simulink model "hdv_hydroelectropowertrain_model"  (R2023b)
settings: Solver=ode1be  StartTime=0.0  StopTime=simulation_length  FixedStep=tsample  MaxStep=tsample
values from neighbouring files (symbols this model uses):
  alpha = 35    [init_model.m]
  Apump = [0 1; 0 0]    [init_model.m]
  available_torque = torque_base+torque_friction_base    [init_model.m]
  Bpump = [0 1]'    [init_model.m]
  btheta_shaft = 2e2    (= 200)    [init_model.m]
  C1 = 10    [init_model.m]
  consumption = [consumption_1, consumption_2, consumption_3, consumption_4,          consumption_5, consumption_6, consumption_7, consumption_8,          consumption_9, consumption_10, consumption_11, consumption_12,          consumption_13, consumption_14, consumption_15, consumption_16          ]    [ic_engine_data.m]
  Cpump = [k 0]    [init_model.m]
  dp_lim = 400    [init_model.m]
  E0 = 3.685    [init_model.m]
  E1 = 0.2156    [init_model.m]
  E2 = 0    [init_model.m]
  E3 = 0    [init_model.m]
  E_1 = -1.031    [init_model.m]
  Elog = -0.05    [init_model.m]
  eta_v_m = 0.98    [init_model.m]
  eta_v_p = 0.97    [init_model.m]
  ki_dp_comp = 1/dp_lim    (= 0.0025)    [init_model.m]
  ki_te_comp = 2/te_lim    [init_model.m]
  kp_ctrl_m = 1    [init_model.m]
  kp_dp_comp = 0.5/dp_lim    (= 0.00125)    [init_model.m]
  kp_te_comp = 1/te_lim    [init_model.m]
  Kpump = acker(Apump,Bpump,poles)    [init_model.m]
  load_blade_enable = 0    [init_model.m]
  Lpump = acker(Apump',Cpump',pole_so)'    [init_model.m]
  M = 125    [init_model.m]
  Ncell = 185    [init_model.m]
  Npump = -1/(Cpump*inv(Apump-Bpump*Kpump)*Bpump)    [init_model.m]
  omega_e_rpm_ref = 1700    [init_model.m]
  omega_l_max_rpm = omega_l_max/(2*pi)*60    (= 50.3075969543)    [init_model.m]
  q1Kalman = tsample^2*1e-2    (= 1e-08)    [init_model.m]
  q2Kalman = tsample^1*1e-1    (= 0.0001)    [init_model.m]
  q3Kalman = 0    [init_model.m]
  Qhr = 400    [init_model.m]
  R0 = 0.015    [init_model.m]
  R1 = 0.015    [init_model.m]
  R_tg = 1.16/2    (= 0.58)    [init_model.m]
  rKalman = 1    [init_model.m]
  rpm_base = [620 700 800 900 1000 1100 1200 1300 1400 1500 1600 1700 1800      1900 2000 2100]    [ic_engine_data.m]
  rpm_consumption = rpm_base    [ic_engine_data.m]
  simulation_length = 245    [init_model.m]
  tau_load = 75e3    (= 75000)    [init_model.m]
  tau_load_max = 1600*41.4    (= 66240)    [init_model.m]
  Tc = tsample    (= 0.001)    [init_model.m]
  torque_base = [max(torque_16_data) max(torque_15_data) max(torque_14_data)      max(torque_13_data) max(torque_12_data) max(torque_11_data)      max(torque_10_data) max(torque_9_data) max(torque_8_data)      max(torque_7_data) max(torque_6_data) max(torque_5_data)      max(torque_4_data) max(torque_3_data) max(torque_2_data)      max(torque_1_data)]    [ic_engine_data.m]
  torque_consumption = torque_reference    [ic_engine_data.m]
  torque_friction_base = -(rpm_base./60*2*pi)*0.25-(rpm_base./60*2*pi).^2*5.2e-4    [ic_engine_data.m]
  tsample = 1e-3    (= 0.001)    [init_model.m]
  v_track1_ref = 8    [init_model.m]
  v_track2_ref = 8    [init_model.m]
  valve_mmorifice_max = 2.75    [init_model.m]
  xv_m_max = 1.2    [init_model.m]
undefined symbols (not defined in the file or in its folder): magnitude
libraries: fl_lib x381, nesl_utility x162, linear_swashplate_ctrl_lib x8, flexshaft_lib x5, bichamber_piston_lib x5, variable_displacement_motor_lib x4, variable_displacement_pump_lib x4, fixed_displacement_pump_lib x4, relief_valve_lib x4, inverse_shuttle_valve_lib x4, hydrostatic_threeway_valve_bichamber_piston_lib x4, hydrostatic_fourway_valve_bichamber_piston_lib x4
(part 5 of 9)

== system hdv_hydroelectropowertrain_model/PR776_powertrain/Hydrostatic_powertrain/driveine_LD2/pressure_charge_system_LD ==
  Hydraulic Flow Rate Sensor : fl_lib/Hydraulic/Hydraulic Sensors/Hydraulic Flow Rate Sensor
  Hydraulic Flow Rate Sensor1 : fl_lib/Hydraulic/Hydraulic Sensors/Hydraulic Flow Rate Sensor
  Hydraulic Pressure Sensor{1..4} (4 alike) : fl_lib/Hydraulic/Hydraulic Sensors/Hydraulic Pressure Sensor
  Hydraulic Reference1 : fl_lib/Hydraulic/Hydraulic Elements/Hydraulic Reference
  Hydraulic Reference2 : fl_lib/Hydraulic/Hydraulic Elements/Hydraulic Reference
  Hydraulic Reference3 : fl_lib/Hydraulic/Hydraulic Elements/Hydraulic Reference
  Mux : Mux  Inputs=2
  PS-Simulink Converter : nesl_utility/PS-Simulink Converter  PhysicalDomain=network_engine_domain  SubClassName=ps_output  LeftPortType=input  RightPortType=output  PseudoPeriodic=off  Frequencies=[]  VectorFormat=1-D array  Unit=l/min  AffineConversion=on
  PS-Simulink Converter{1..3,5} (4 alike) : nesl_utility/PS-Simulink Converter  PhysicalDomain=network_engine_domain  SubClassName=ps_output  LeftPortType=input  RightPortType=output  PseudoPeriodic=off  Frequencies=[]  VectorFormat=1-D array  Unit=bar  AffineConversion=on
  PS-Simulink Converter4 : nesl_utility/PS-Simulink Converter  PhysicalDomain=network_engine_domain  SubClassName=ps_output  LeftPortType=input  RightPortType=output  PseudoPeriodic=off  Frequencies=[]  VectorFormat=1-D array  Unit=l/min  AffineConversion=on
  Scope1 : Scope  NumInputPorts=2
  Scope2 : Scope  NumInputPorts=2
  Scope3 : Scope  NumInputPorts=2
  Subsystem : Subsystem
  hydro_check_valve1 : Subsystem
      settings: PortSchema="{\"entries\":[{\"content\":{\"sides\":[{\"content\":{\"connectorIds\":[]},\"type\":\"ConnectorPlacement.EquallySpacedRectSide\",\"uuid\":\"a69fbb91-2279-4dfd-af6f-16497d5f1538\"},{\"content\":{\"connectorIds\":[],\"side\":\"RIGHT\"},\"type\":\"ConnectorPlacement.EquallySpacedRectSide\",\"uuid\":\"52e95d44-b7af-4ccc-8556-a2abd2e724e0\"},{\"content\":{\"connectorIds\":[\"LConn1\"],\"side\":\"TOP\"},\"type\":\"ConnectorPlacement.EquallySpacedRectSide\",\"uuid\":\"2d8c071e-4cd0-4b83-8d45-c175cb858754\"},{\"content\":{\"connectorIds\":[\"RConn1\"],\"side\":\"BOTTOM\"},\"type\":\"ConnectorPlacement.EquallySpacedRectSide\",\"uuid\":\"1baec9dc-757c-4f21-904a-6fc08de72ce1\"}]},\"type\":\"ConnectorPlacement.EquallySpacedConnector\",\"uuid\":\"76990e53-6cb0-4bfe-8c9e-427c41b785f2\"}],\"packageUris\":[\"http://schema.mathworks.com/mf0/Connector/19700101\"],\"version\":\"1.0\"}"
  hydro_check_valve2 : Subsystem
      settings: PortSchema="{\"entries\":[{\"content\":{\"sides\":[{\"content\":{\"connectorIds\":[]},\"type\":\"ConnectorPlacement.EquallySpacedRectSide\",\"uuid\":\"a69fbb91-2279-4dfd-af6f-16497d5f1538\"},{\"content\":{\"connectorIds\":[],\"side\":\"RIGHT\"},\"type\":\"ConnectorPlacement.EquallySpacedRectSide\",\"uuid\":\"52e95d44-b7af-4ccc-8556-a2abd2e724e0\"},{\"content\":{\"connectorIds\":[\"LConn1\"],\"side\":\"TOP\"},\"type\":\"ConnectorPlacement.EquallySpacedRectSide\",\"uuid\":\"2d8c071e-4cd0-4b83-8d45-c175cb858754\"},{\"content\":{\"connectorIds\":[\"RConn1\"],\"side\":\"BOTTOM\"},\"type\":\"ConnectorPlacement.EquallySpacedRectSide\",\"uuid\":\"1baec9dc-757c-4f21-904a-6fc08de72ce1\"}]},\"type\":\"ConnectorPlacement.EquallySpacedConnector\",\"uuid\":\"76990e53-6cb0-4bfe-8c9e-427c41b785f2\"}],\"packageUris\":[\"http://schema.mathworks.com/mf0/Connector/19700101\"],\"version\":\"1.0\"}"
  inverse shuttle valve : inverse_shuttle_valve_lib/inverse shuttle valve  pnom=32 bar  dp_crack=0 bar  dp_reg=0 bar  x_rv_max=2 mm  a0=(2*pi*10)^2 1/s^2  a1=2*2*pi*10 1/s  leak=5e-12 m^3/s/Pa  qA_specify=off  qA_priority=None  qA=0 m^3/s  qA_nominal_specify=off  qA_nominal_unit=m^3/s  qA_nominal_value=1  qB_specify=off  qB_priority=None  qB=0 m^3/s  qB_nominal_specify=off  qB_nominal_unit=m^3/s  qB_nominal_value=1  qP_specify=off  qP_priority=None  qP=0 m^3/s  qP_nominal_specify=off  qP_nominal_unit=m^3/s  qP_nominal_value=1  dp_specify=off  dp_priority=None  dp=0 Pa  dp_nominal_specify=off  dp_nominal_unit=Pa  dp_nominal_value=1  dpAP_specify=off  dpAP_priority=None  dpAP=0 Pa  dpAP_nominal_specify=off  dpAP_nominal_unit=Pa  dpAP_nominal_value=1  dpBP_specify=off  dpBP_priority=None  dpBP=0 Pa  dpBP_nominal_specify=off  dpBP_nominal_unit=Pa  dpBP_nominal_value=1  x_rv_AP_specify=off  x_rv_AP_priority=None  x_rv_AP=0 m  x_rv_AP_nominal_specify=off  x_rv_AP_nominal_unit=m  x_rv_AP_nominal_value=1  x_rv_BP_specify=off  x_rv_BP_priority=None  x_rv_BP=0 m  x_rv_BP_nominal_specify=off  x_rv_BP_nominal_unit=m  x_rv_BP_nominal_value=1  x_rv_AP_flt_specify=off  x_rv_AP_flt_priority=None  x_rv_AP_flt=0 m  x_rv_AP_flt_nominal_specify=off  x_rv_AP_flt_nominal_unit=m  x_rv_AP_flt_nominal_value=1  x_rv_BP_flt_specify=off  x_rv_BP_flt_priority=None  x_rv_BP_flt=0 m  x_rv_BP_flt_nominal_specify=off  x_rv_BP_flt_nominal_unit=m  x_rv_BP_flt_nominal_value=1
      settings: InternalSimscapePortConfiguration="{\"Bottom\":[],\"Left\":[{\"id\":\"cA\",\"label\":\"cA\",\"type\":\"foundation.hydraulic.hydraulic\"},{\"id\":\"cB\",\"label\":\"cB\",\"type\":\"foundation.hydraulic.hydraulic\"}],\"Right\":[{\"id\":\"cP\",\"label\":\"cP\",\"type\":\"foundation.hydraulic.hydraulic\"}],\"Top\":[]}"
  A : PMIOPort  Side=Left
  B : PMIOPort  Port=2  Side=Right
  D : PMIOPort  Port=3  Side=Right
  wires:
  PS-Simulink Converter2/1 -> Mux/2  "pA"
  PS-Simulink Converter1/1 -> Mux/1  "pB"
  Mux/1 -> Scope1/1
  PS-Simulink Converter/1 -> Scope2/1, Scope1/2  "qcharge"
  PS-Simulink Converter3/1 -> Scope2/2  "pCharge"
  PS-Simulink Converter4/1 -> Scope3/1  "qT_ishuttle"
  PS-Simulink Converter5/1 -> Scope3/2  "dp"
  connections:
  inverse shuttle valve/RConn1 -- Hydraulic Flow Rate Sensor1/LConn1
  hydro_check_valve2/LConn1 -- Hydraulic Flow Rate Sensor/RConn2 -- hydro_check_valve1/LConn1
  hydro_check_valve1/RConn1 -- inverse shuttle valve/LConn1 -- A/RConn1 -- Hydraulic Pressure Sensor2/LConn1 -- Hydraulic Pressure Sensor4/LConn1
  hydro_check_valve2/RConn1 -- inverse shuttle valve/LConn2 -- B/RConn1 -- Hydraulic Pressure Sensor1/LConn1 -- Hydraulic Pressure Sensor4/RConn1
  Hydraulic Pressure Sensor2/RConn1 -- Hydraulic Reference1/LConn1 -- Hydraulic Pressure Sensor1/RConn1
  Hydraulic Pressure Sensor1/RConn2 -- PS-Simulink Converter1/LConn1
  Hydraulic Pressure Sensor2/RConn2 -- PS-Simulink Converter2/LConn1
  Hydraulic Flow Rate Sensor/RConn1 -- PS-Simulink Converter/LConn1
  Hydraulic Pressure Sensor3/LConn1 -- Subsystem/RConn1 -- Hydraulic Flow Rate Sensor/LConn1
  Subsystem/LConn1 -- D/RConn1
  Hydraulic Pressure Sensor3/RConn2 -- PS-Simulink Converter3/LConn1
  Hydraulic Reference2/LConn1 -- Hydraulic Pressure Sensor3/RConn1
  Hydraulic Flow Rate Sensor1/RConn2 -- Hydraulic Reference3/LConn1
  Hydraulic Flow Rate Sensor1/RConn1 -- PS-Simulink Converter4/LConn1
  PS-Simulink Converter5/LConn1 -- Hydraulic Pressure Sensor4/RConn2

== system hdv_hydroelectropowertrain_model/PR776_powertrain/Hydrostatic_powertrain/driveine_LD2/vd_ctrl_motor_LD ==
  vd_ref : Inport
  Linear swashplate ctrl2 : linear_swashplate_ctrl_lib/Linear swashplate ctrl  Commented=on  a12=1 1/s  b2=1 1/m/s  k1=100 m  k2=20.5 m  N=5 m  kv=20  xv_specify=off  xv_priority=None  xv=0 m  xv_nominal_specify=off  xv_nominal_unit=m  xv_nominal_value=1  D1_specify=off  D1_priority=None  D1=0  D1_nominal_specify=off  D1_nominal_unit=1  D1_nominal_value=1  D2_specify=off  D2_priority=None  D2=0  D2_nominal_specify=off  D2_nominal_unit=1  D2_nominal_value=1
      settings: InternalSimscapePortConfiguration="{\"Bottom\":[],\"Left\":[{\"id\":\"D_ref\",\"label\":\"Dref\",\"type\":\"input\"}],\"Right\":[{\"id\":\"Dout\",\"label\":\"Dout\",\"type\":\"output\"}],\"Top\":[]}"
  PS-Simulink Converter : nesl_utility/PS-Simulink Converter  PhysicalDomain=network_engine_domain  SubClassName=ps_output  LeftPortType=input  RightPortType=output  PseudoPeriodic=off  Frequencies=[]  VectorFormat=1-D array  Unit=inherit  AffineConversion=off
  Scope : Scope  NumInputPorts=2
  Simulink-PS Converter3 : nesl_utility/Simulink-PS Converter  Commented=on  PhysicalDomain=network_engine_domain  SubClassName=ps_input  LeftPortType=input  RightPortType=output  PseudoPeriodic=off  Frequencies=[]  NoiseDistribution=none  NoiseParameters=[]  Unit=1  AffineConversion=off  FilteringAndDerivatives=provide  SimscapeFilterOrder=1  InputFilterTimeConstant=0.001  UdotUserProvided=0
  hose3 : Subsystem
  servo motor LD : Subsystem
  vd : PMIOPort  Side=Right
  pS : PMIOPort  Port=2  Side=Left
  pT : PMIOPort  Port=3  Side=Left
  wires:
  vd_ref/1 -> Simulink-PS Converter3/1, Scope/1, servo motor LD/1(displacement reference pu)
  PS-Simulink Converter/1 -> Scope/2
  connections:
  vd/RConn1 -- PS-Simulink Converter/LConn1 -- servo motor LD/RConn1
  hose3/RConn2 -- servo motor LD/LConn2
  hose3/RConn1 -- servo motor LD/LConn1
  pT/RConn1 -- hose3/LConn2
  pS/RConn1 -- hose3/LConn1
  Simulink-PS Converter3/RConn1 -- Linear swashplate ctrl2/LConn1

== system hdv_hydroelectropowertrain_model/PR776_powertrain/Hydrostatic_powertrain/driveine_LD2/vd_ctrl_pump_LD ==
  vd_ref : Inport
  Linear swashplate ctrl2 : linear_swashplate_ctrl_lib/Linear swashplate ctrl  Commented=on  a12=1 1/s  b2=1 1/m/s  k1=100 m  k2=20.5 m  N=5 m  kv=20  xv_specify=off  xv_priority=None  xv=0 m  xv_nominal_specify=off  xv_nominal_unit=m  xv_nominal_value=1  D1_specify=off  D1_priority=None  D1=0  D1_nominal_specify=off  D1_nominal_unit=1  D1_nominal_value=1  D2_specify=off  D2_priority=None  D2=0  D2_nominal_specify=off  D2_nominal_unit=1  D2_nominal_value=1
      settings: InternalSimscapePortConfiguration="{\"Bottom\":[],\"Left\":[{\"id\":\"D_ref\",\"label\":\"Dref\",\"type\":\"input\"}],\"Right\":[{\"id\":\"Dout\",\"label\":\"Dout\",\"type\":\"output\"}],\"Top\":[]}"
  Simulink-PS Converter3 : nesl_utility/Simulink-PS Converter  Commented=on  PhysicalDomain=network_engine_domain  SubClassName=ps_input  LeftPortType=input  RightPortType=output  PseudoPeriodic=off  Frequencies=[]  NoiseDistribution=none  NoiseParameters=[]  Unit=1  AffineConversion=off  FilteringAndDerivatives=provide  SimscapeFilterOrder=1  InputFilterTimeConstant=0.001  UdotUserProvided=0
  hose3 : Subsystem
  servo pump RD : Subsystem
  vd : PMIOPort  Side=Right
  pS : PMIOPort  Port=2  Side=Left
  pT : PMIOPort  Port=3  Side=Left
  wires:
  vd_ref/1 -> servo pump RD/1(displacement reference pu), Simulink-PS Converter3/1
  connections:
  servo pump RD/RConn1 -- vd/RConn1
  Simulink-PS Converter3/RConn1 -- Linear swashplate ctrl2/LConn1
  servo pump RD/LConn2 -- hose3/RConn2
  servo pump RD/LConn1 -- hose3/RConn1
  pS/RConn1 -- hose3/LConn1
  pT/RConn1 -- hose3/LConn2

== system hdv_hydroelectropowertrain_model/PR776_powertrain/Hydrostatic_powertrain/driveine_RD1/pressure_charge_system_RD ==
  Hydraulic Flow Rate Sensor : fl_lib/Hydraulic/Hydraulic Sensors/Hydraulic Flow Rate Sensor
  Hydraulic Flow Rate Sensor1 : fl_lib/Hydraulic/Hydraulic Sensors/Hydraulic Flow Rate Sensor
  Hydraulic Pressure Sensor{1..4} (4 alike) : fl_lib/Hydraulic/Hydraulic Sensors/Hydraulic Pressure Sensor
  Hydraulic Reference1 : fl_lib/Hydraulic/Hydraulic Elements/Hydraulic Reference
  Hydraulic Reference2 : fl_lib/Hydraulic/Hydraulic Elements/Hydraulic Reference
  Hydraulic Reference3 : fl_lib/Hydraulic/Hydraulic Elements/Hydraulic Reference
  Mux : Mux  Inputs=2
  PS-Simulink Converter : nesl_utility/PS-Simulink Converter  PhysicalDomain=network_engine_domain  SubClassName=ps_output  LeftPortType=input  RightPortType=output  PseudoPeriodic=off  Frequencies=[]  VectorFormat=1-D array  Unit=l/min  AffineConversion=on
  PS-Simulink Converter{1..3,5} (4 alike) : nesl_utility/PS-Simulink Converter  PhysicalDomain=network_engine_domain  SubClassName=ps_output  LeftPortType=input  RightPortType=output  PseudoPeriodic=off  Frequencies=[]  VectorFormat=1-D array  Unit=bar  AffineConversion=on
  PS-Simulink Converter4 : nesl_utility/PS-Simulink Converter  PhysicalDomain=network_engine_domain  SubClassName=ps_output  LeftPortType=input  RightPortType=output  PseudoPeriodic=off  Frequencies=[]  VectorFormat=1-D array  Unit=l/min  AffineConversion=on
  Scope1 : Scope  NumInputPorts=2
  Scope2 : Scope  NumInputPorts=2
  Subsystem : Subsystem
  hydro_check_valve1 : Subsystem
      settings: PortSchema="{\"entries\":[{\"content\":{\"sides\":[{\"content\":{\"connectorIds\":[]},\"type\":\"ConnectorPlacement.EquallySpacedRectSide\",\"uuid\":\"a69fbb91-2279-4dfd-af6f-16497d5f1538\"},{\"content\":{\"connectorIds\":[],\"side\":\"RIGHT\"},\"type\":\"ConnectorPlacement.EquallySpacedRectSide\",\"uuid\":\"52e95d44-b7af-4ccc-8556-a2abd2e724e0\"},{\"content\":{\"connectorIds\":[\"LConn1\"],\"side\":\"TOP\"},\"type\":\"ConnectorPlacement.EquallySpacedRectSide\",\"uuid\":\"2d8c071e-4cd0-4b83-8d45-c175cb858754\"},{\"content\":{\"connectorIds\":[\"RConn1\"],\"side\":\"BOTTOM\"},\"type\":\"ConnectorPlacement.EquallySpacedRectSide\",\"uuid\":\"1baec9dc-757c-4f21-904a-6fc08de72ce1\"}]},\"type\":\"ConnectorPlacement.EquallySpacedConnector\",\"uuid\":\"76990e53-6cb0-4bfe-8c9e-427c41b785f2\"}],\"packageUris\":[\"http://schema.mathworks.com/mf0/Connector/19700101\"],\"version\":\"1.0\"}"
  hydro_check_valve2 : Subsystem
      settings: PortSchema="{\"entries\":[{\"content\":{\"sides\":[{\"content\":{\"connectorIds\":[]},\"type\":\"ConnectorPlacement.EquallySpacedRectSide\",\"uuid\":\"a69fbb91-2279-4dfd-af6f-16497d5f1538\"},{\"content\":{\"connectorIds\":[],\"side\":\"RIGHT\"},\"type\":\"ConnectorPlacement.EquallySpacedRectSide\",\"uuid\":\"52e95d44-b7af-4ccc-8556-a2abd2e724e0\"},{\"content\":{\"connectorIds\":[\"LConn1\"],\"side\":\"TOP\"},\"type\":\"ConnectorPlacement.EquallySpacedRectSide\",\"uuid\":\"2d8c071e-4cd0-4b83-8d45-c175cb858754\"},{\"content\":{\"connectorIds\":[\"RConn1\"],\"side\":\"BOTTOM\"},\"type\":\"ConnectorPlacement.EquallySpacedRectSide\",\"uuid\":\"1baec9dc-757c-4f21-904a-6fc08de72ce1\"}]},\"type\":\"ConnectorPlacement.EquallySpacedConnector\",\"uuid\":\"76990e53-6cb0-4bfe-8c9e-427c41b785f2\"}],\"packageUris\":[\"http://schema.mathworks.com/mf0/Connector/19700101\"],\"version\":\"1.0\"}"
  inverse shuttle valve : inverse_shuttle_valve_lib/inverse shuttle valve  pnom=32 bar  dp_crack=0 bar  dp_reg=0 bar  x_rv_max=2 mm  a0=(2*pi*10)^2 1/s^2  a1=2*2*pi*10 1/s  leak=5e-12 m^3/s/Pa  qA_specify=off  qA_priority=None  qA=0 m^3/s  qA_nominal_specify=off  qA_nominal_unit=m^3/s  qA_nominal_value=1  qB_specify=off  qB_priority=None  qB=0 m^3/s  qB_nominal_specify=off  qB_nominal_unit=m^3/s  qB_nominal_value=1  qP_specify=off  qP_priority=None  qP=0 m^3/s  qP_nominal_specify=off  qP_nominal_unit=m^3/s  qP_nominal_value=1  dp_specify=off  dp_priority=None  dp=0 Pa  dp_nominal_specify=off  dp_nominal_unit=Pa  dp_nominal_value=1  dpAP_specify=off  dpAP_priority=None  dpAP=0 Pa  dpAP_nominal_specify=off  dpAP_nominal_unit=Pa  dpAP_nominal_value=1  dpBP_specify=off  dpBP_priority=None  dpBP=0 Pa  dpBP_nominal_specify=off  dpBP_nominal_unit=Pa  dpBP_nominal_value=1  x_rv_AP_specify=off  x_rv_AP_priority=None  x_rv_AP=0 m  x_rv_AP_nominal_specify=off  x_rv_AP_nominal_unit=m  x_rv_AP_nominal_value=1  x_rv_BP_specify=off  x_rv_BP_priority=None  x_rv_BP=0 m  x_rv_BP_nominal_specify=off  x_rv_BP_nominal_unit=m  x_rv_BP_nominal_value=1  x_rv_AP_flt_specify=off  x_rv_AP_flt_priority=None  x_rv_AP_flt=0 m  x_rv_AP_flt_nominal_specify=off  x_rv_AP_flt_nominal_unit=m  x_rv_AP_flt_nominal_value=1  x_rv_BP_flt_specify=off  x_rv_BP_flt_priority=None  x_rv_BP_flt=0 m  x_rv_BP_flt_nominal_specify=off  x_rv_BP_flt_nominal_unit=m  x_rv_BP_flt_nominal_value=1
      settings: InternalSimscapePortConfiguration="{\"Bottom\":[],\"Left\":[{\"id\":\"cA\",\"label\":\"cA\",\"type\":\"foundation.hydraulic.hydraulic\"},{\"id\":\"cB\",\"label\":\"cB\",\"type\":\"foundation.hydraulic.hydraulic\"}],\"Right\":[{\"id\":\"cP\",\"label\":\"cP\",\"type\":\"foundation.hydraulic.hydraulic\"}],\"Top\":[]}"
  qt_ishuttle/dp : Scope  NumInputPorts=2
  A : PMIOPort  Side=Left
  B : PMIOPort  Port=2  Side=Right
  D : PMIOPort  Port=3  Side=Right
  wires:
  PS-Simulink Converter2/1 -> Mux/2  "pA"
  PS-Simulink Converter1/1 -> Mux/1  "pB"
  Mux/1 -> Scope1/1
  PS-Simulink Converter/1 -> Scope1/2, Scope2/1  "qcharge"
  PS-Simulink Converter3/1 -> Scope2/2  "pCharge"
  PS-Simulink Converter4/1 -> qt_ishuttle/dp/1  "qt_ishuttle"
  PS-Simulink Converter5/1 -> qt_ishuttle/dp/2  "dp"
  connections:
  hydro_check_valve2/LConn1 -- Hydraulic Flow Rate Sensor/RConn2 -- hydro_check_valve1/LConn1
  A/RConn1 -- Hydraulic Pressure Sensor4/LConn1 -- inverse shuttle valve/LConn1 -- hydro_check_valve1/RConn1 -- Hydraulic Pressure Sensor2/LConn1
  B/RConn1 -- Hydraulic Pressure Sensor4/RConn1 -- inverse shuttle valve/LConn2 -- hydro_check_valve2/RConn1 -- Hydraulic Pressure Sensor1/LConn1
  Hydraulic Pressure Sensor2/RConn1 -- Hydraulic Reference1/LConn1 -- Hydraulic Pressure Sensor1/RConn1
  Hydraulic Pressure Sensor1/RConn2 -- PS-Simulink Converter1/LConn1
  Hydraulic Pressure Sensor2/RConn2 -- PS-Simulink Converter2/LConn1
  Hydraulic Flow Rate Sensor/RConn1 -- PS-Simulink Converter/LConn1
  Hydraulic Pressure Sensor3/LConn1 -- Subsystem/RConn1 -- Hydraulic Flow Rate Sensor/LConn1
  Subsystem/LConn1 -- D/RConn1
  Hydraulic Pressure Sensor3/RConn2 -- PS-Simulink Converter3/LConn1
  Hydraulic Reference2/LConn1 -- Hydraulic Pressure Sensor3/RConn1
  Hydraulic Flow Rate Sensor1/RConn2 -- Hydraulic Reference3/LConn1
  Hydraulic Flow Rate Sensor1/RConn1 -- PS-Simulink Converter4/LConn1
  PS-Simulink Converter5/LConn1 -- Hydraulic Pressure Sensor4/RConn2
  inverse shuttle valve/RConn1 -- Hydraulic Flow Rate Sensor1/LConn1

== system hdv_hydroelectropowertrain_model/PR776_powertrain/Hydrostatic_powertrain/driveine_RD1/vd_ctrl_motor_RD ==
  vd_ref : Inport
  Linear swashplate ctrl2 : linear_swashplate_ctrl_lib/Linear swashplate ctrl  Commented=on  a12=1 1/s  b2=1 1/m/s  k1=100 m  k2=20.5 m  N=5 m  kv=20  xv_specify=off  xv_priority=None  xv=0 m  xv_nominal_specify=off  xv_nominal_unit=m  xv_nominal_value=1  D1_specify=off  D1_priority=None  D1=0  D1_nominal_specify=off  D1_nominal_unit=1  D1_nominal_value=1  D2_specify=off  D2_priority=None  D2=0  D2_nominal_specify=off  D2_nominal_unit=1  D2_nominal_value=1
      settings: InternalSimscapePortConfiguration="{\"Bottom\":[],\"Left\":[{\"id\":\"D_ref\",\"label\":\"Dref\",\"type\":\"input\"}],\"Right\":[{\"id\":\"Dout\",\"label\":\"Dout\",\"type\":\"output\"}],\"Top\":[]}"
  PS-Simulink Converter : nesl_utility/PS-Simulink Converter  PhysicalDomain=network_engine_domain  SubClassName=ps_output  LeftPortType=input  RightPortType=output  PseudoPeriodic=off  Frequencies=[]  VectorFormat=1-D array  Unit=inherit  AffineConversion=off
  Scope : Scope  NumInputPorts=2
  Simulink-PS Converter3 : nesl_utility/Simulink-PS Converter  Commented=on  PhysicalDomain=network_engine_domain  SubClassName=ps_input  LeftPortType=input  RightPortType=output  PseudoPeriodic=off  Frequencies=[]  NoiseDistribution=none  NoiseParameters=[]  Unit=1  AffineConversion=off  FilteringAndDerivatives=provide  SimscapeFilterOrder=1  InputFilterTimeConstant=0.001  UdotUserProvided=0
  hose3 : Subsystem
  servo motor LD : Subsystem
  vd : PMIOPort  Side=Right
  pS : PMIOPort  Port=2  Side=Left
  pT : PMIOPort  Port=3  Side=Left
  wires:
  vd_ref/1 -> Scope/1, Simulink-PS Converter3/1, servo motor LD/1(displacement reference pu)
  PS-Simulink Converter/1 -> Scope/2
  connections:
  hose3/RConn2 -- servo motor LD/LConn2
  hose3/RConn1 -- servo motor LD/LConn1
  pS/RConn1 -- hose3/LConn1
  pT/RConn1 -- hose3/LConn2
  Simulink-PS Converter3/RConn1 -- Linear swashplate ctrl2/LConn1
  servo motor LD/RConn1 -- PS-Simulink Converter/LConn1 -- vd/RConn1

== system hdv_hydroelectropowertrain_model/PR776_powertrain/Hydrostatic_powertrain/driveine_RD1/vd_ctrl_pump_RD ==
  vd_ref : Inport
  Linear swashplate ctrl2 : linear_swashplate_ctrl_lib/Linear swashplate ctrl  Commented=on  a12=1 1/s  b2=1 1/m/s  k1=100 m  k2=20.5 m  N=5 m  kv=20  xv_specify=off  xv_priority=None  xv=0 m  xv_nominal_specify=off  xv_nominal_unit=m  xv_nominal_value=1  D1_specify=off  D1_priority=None  D1=0  D1_nominal_specify=off  D1_nominal_unit=1  D1_nominal_value=1  D2_specify=off  D2_priority=None  D2=0  D2_nominal_specify=off  D2_nominal_unit=1  D2_nominal_value=1
      settings: InternalSimscapePortConfiguration="{\"Bottom\":[],\"Left\":[{\"id\":\"D_ref\",\"label\":\"Dref\",\"type\":\"input\"}],\"Right\":[{\"id\":\"Dout\",\"label\":\"Dout\",\"type\":\"output\"}],\"Top\":[]}"
  Simulink-PS Converter3 : nesl_utility/Simulink-PS Converter  Commented=on  PhysicalDomain=network_engine_domain  SubClassName=ps_input  LeftPortType=input  RightPortType=output  PseudoPeriodic=off  Frequencies=[]  NoiseDistribution=none  NoiseParameters=[]  Unit=1  AffineConversion=off  FilteringAndDerivatives=provide  SimscapeFilterOrder=1  InputFilterTimeConstant=0.001  UdotUserProvided=0
  hose3 : Subsystem
  servo pump RD : Subsystem
  vd : PMIOPort  Side=Right
  pS : PMIOPort  Port=2  Side=Left
  pT : PMIOPort  Port=3  Side=Left
  wires:
  vd_ref/1 -> servo pump RD/1(displacement reference pu), Simulink-PS Converter3/1
  connections:
  servo pump RD/LConn2 -- hose3/RConn2
  servo pump RD/LConn1 -- hose3/RConn1
  pS/RConn1 -- hose3/LConn1
  pT/RConn1 -- hose3/LConn2
  Simulink-PS Converter3/RConn1 -- Linear swashplate ctrl2/LConn1
  servo pump RD/RConn1 -- vd/RConn1

== system hdv_hydroelectropowertrain_model/PR776_powertrain/Hydrostatic_powertrain/driveline_RD2/pressure_charge_system_RD ==
  Hydraulic Flow Rate Sensor : fl_lib/Hydraulic/Hydraulic Sensors/Hydraulic Flow Rate Sensor
  Hydraulic Flow Rate Sensor1 : fl_lib/Hydraulic/Hydraulic Sensors/Hydraulic Flow Rate Sensor
  Hydraulic Pressure Sensor{1..4} (4 alike) : fl_lib/Hydraulic/Hydraulic Sensors/Hydraulic Pressure Sensor
  Hydraulic Reference1 : fl_lib/Hydraulic/Hydraulic Elements/Hydraulic Reference
  Hydraulic Reference2 : fl_lib/Hydraulic/Hydraulic Elements/Hydraulic Reference
  Hydraulic Reference3 : fl_lib/Hydraulic/Hydraulic Elements/Hydraulic Reference
  Mux : Mux  Inputs=2
  PS-Simulink Converter : nesl_utility/PS-Simulink Converter  PhysicalDomain=network_engine_domain  SubClassName=ps_output  LeftPortType=input  RightPortType=output  PseudoPeriodic=off  Frequencies=[]  VectorFormat=1-D array  Unit=l/min  AffineConversion=on
  PS-Simulink Converter{1..3,5} (4 alike) : nesl_utility/PS-Simulink Converter  PhysicalDomain=network_engine_domain  SubClassName=ps_output  LeftPortType=input  RightPortType=output  PseudoPeriodic=off  Frequencies=[]  VectorFormat=1-D array  Unit=bar  AffineConversion=on
  PS-Simulink Converter4 : nesl_utility/PS-Simulink Converter  PhysicalDomain=network_engine_domain  SubClassName=ps_output  LeftPortType=input  RightPortType=output  PseudoPeriodic=off  Frequencies=[]  VectorFormat=1-D array  Unit=l/min  AffineConversion=on
  Scope1 : Scope  NumInputPorts=2
  Scope2 : Scope  NumInputPorts=2
  Subsystem : Subsystem
  hydro_check_valve1 : Subsystem
      settings: PortSchema="{\"entries\":[{\"content\":{\"sides\":[{\"content\":{\"connectorIds\":[]},\"type\":\"ConnectorPlacement.EquallySpacedRectSide\",\"uuid\":\"a69fbb91-2279-4dfd-af6f-16497d5f1538\"},{\"content\":{\"connectorIds\":[],\"side\":\"RIGHT\"},\"type\":\"ConnectorPlacement.EquallySpacedRectSide\",\"uuid\":\"52e95d44-b7af-4ccc-8556-a2abd2e724e0\"},{\"content\":{\"connectorIds\":[\"LConn1\"],\"side\":\"TOP\"},\"type\":\"ConnectorPlacement.EquallySpacedRectSide\",\"uuid\":\"2d8c071e-4cd0-4b83-8d45-c175cb858754\"},{\"content\":{\"connectorIds\":[\"RConn1\"],\"side\":\"BOTTOM\"},\"type\":\"ConnectorPlacement.EquallySpacedRectSide\",\"uuid\":\"1baec9dc-757c-4f21-904a-6fc08de72ce1\"}]},\"type\":\"ConnectorPlacement.EquallySpacedConnector\",\"uuid\":\"76990e53-6cb0-4bfe-8c9e-427c41b785f2\"}],\"packageUris\":[\"http://schema.mathworks.com/mf0/Connector/19700101\"],\"version\":\"1.0\"}"
  hydro_check_valve2 : Subsystem
      settings: PortSchema="{\"entries\":[{\"content\":{\"sides\":[{\"content\":{\"connectorIds\":[]},\"type\":\"ConnectorPlacement.EquallySpacedRectSide\",\"uuid\":\"a69fbb91-2279-4dfd-af6f-16497d5f1538\"},{\"content\":{\"connectorIds\":[],\"side\":\"RIGHT\"},\"type\":\"ConnectorPlacement.EquallySpacedRectSide\",\"uuid\":\"52e95d44-b7af-4ccc-8556-a2abd2e724e0\"},{\"content\":{\"connectorIds\":[\"LConn1\"],\"side\":\"TOP\"},\"type\":\"ConnectorPlacement.EquallySpacedRectSide\",\"uuid\":\"2d8c071e-4cd0-4b83-8d45-c175cb858754\"},{\"content\":{\"connectorIds\":[\"RConn1\"],\"side\":\"BOTTOM\"},\"type\":\"ConnectorPlacement.EquallySpacedRectSide\",\"uuid\":\"1baec9dc-757c-4f21-904a-6fc08de72ce1\"}]},\"type\":\"ConnectorPlacement.EquallySpacedConnector\",\"uuid\":\"76990e53-6cb0-4bfe-8c9e-427c41b785f2\"}],\"packageUris\":[\"http://schema.mathworks.com/mf0/Connector/19700101\"],\"version\":\"1.0\"}"
  inverse shuttle valve : inverse_shuttle_valve_lib/inverse shuttle valve  pnom=32 bar  dp_crack=0 bar  dp_reg=0 bar  x_rv_max=2 mm  a0=(2*pi*10)^2 1/s^2  a1=2*2*pi*10 1/s  leak=5e-12 m^3/s/Pa  qA_specify=off  qA_priority=None  qA=0 m^3/s  qA_nominal_specify=off  qA_nominal_unit=m^3/s  qA_nominal_value=1  qB_specify=off  qB_priority=None  qB=0 m^3/s  qB_nominal_specify=off  qB_nominal_unit=m^3/s  qB_nominal_value=1  qP_specify=off  qP_priority=None  qP=0 m^3/s  qP_nominal_specify=off  qP_nominal_unit=m^3/s  qP_nominal_value=1  dp_specify=off  dp_priority=None  dp=0 Pa  dp_nominal_specify=off  dp_nominal_unit=Pa  dp_nominal_value=1  dpAP_specify=off  dpAP_priority=None  dpAP=0 Pa  dpAP_nominal_specify=off  dpAP_nominal_unit=Pa  dpAP_nominal_value=1  dpBP_specify=off  dpBP_priority=None  dpBP=0 Pa  dpBP_nominal_specify=off  dpBP_nominal_unit=Pa  dpBP_nominal_value=1  x_rv_AP_specify=off  x_rv_AP_priority=None  x_rv_AP=0 m  x_rv_AP_nominal_specify=off  x_rv_AP_nominal_unit=m  x_rv_AP_nominal_value=1  x_rv_BP_specify=off  x_rv_BP_priority=None  x_rv_BP=0 m  x_rv_BP_nominal_specify=off  x_rv_BP_nominal_unit=m  x_rv_BP_nominal_value=1  x_rv_AP_flt_specify=off  x_rv_AP_flt_priority=None  x_rv_AP_flt=0 m  x_rv_AP_flt_nominal_specify=off  x_rv_AP_flt_nominal_unit=m  x_rv_AP_flt_nominal_value=1  x_rv_BP_flt_specify=off  x_rv_BP_flt_priority=None  x_rv_BP_flt=0 m  x_rv_BP_flt_nominal_specify=off  x_rv_BP_flt_nominal_unit=m  x_rv_BP_flt_nominal_value=1
      settings: InternalSimscapePortConfiguration="{\"Bottom\":[],\"Left\":[{\"id\":\"cA\",\"label\":\"cA\",\"type\":\"foundation.hydraulic.hydraulic\"},{\"id\":\"cB\",\"label\":\"cB\",\"type\":\"foundation.hydraulic.hydraulic\"}],\"Right\":[{\"id\":\"cP\",\"label\":\"cP\",\"type\":\"foundation.hydraulic.hydraulic\"}],\"Top\":[]}"
  qt_ishuttle/dp : Scope  NumInputPorts=2
  A : PMIOPort  Side=Left
  B : PMIOPort  Port=2  Side=Right
  D : PMIOPort  Port=3  Side=Right
  wires:
  PS-Simulink Converter5/1 -> qt_ishuttle/dp/2  "dp"
  PS-Simulink Converter4/1 -> qt_ishuttle/dp/1  "qt_ishuttle"
  PS-Simulink Converter3/1 -> Scope2/2  "pCharge"
  PS-Simulink Converter/1 -> Scope2/1, Scope1/2  "qcharge"
  Mux/1 -> Scope1/1
  PS-Simulink Converter1/1 -> Mux/1  "pB"
  PS-Simulink Converter2/1 -> Mux/2  "pA"
  connections:
  inverse shuttle valve/RConn1 -- Hydraulic Flow Rate Sensor1/LConn1
  PS-Simulink Converter5/LConn1 -- Hydraulic Pressure Sensor4/RConn2
  Hydraulic Flow Rate Sensor1/RConn1 -- PS-Simulink Converter4/LConn1
  Hydraulic Flow Rate Sensor1/RConn2 -- Hydraulic Reference3/LConn1
  Hydraulic Reference2/LConn1 -- Hydraulic Pressure Sensor3/RConn1
  Hydraulic Pressure Sensor3/RConn2 -- PS-Simulink Converter3/LConn1
  Subsystem/LConn1 -- D/RConn1
  Hydraulic Flow Rate Sensor/LConn1 -- Subsystem/RConn1 -- Hydraulic Pressure Sensor3/LConn1
  Hydraulic Flow Rate Sensor/RConn1 -- PS-Simulink Converter/LConn1
  Hydraulic Pressure Sensor2/RConn2 -- PS-Simulink Converter2/LConn1
  Hydraulic Pressure Sensor1/RConn2 -- PS-Simulink Converter1/LConn1
  Hydraulic Pressure Sensor1/RConn1 -- Hydraulic Reference1/LConn1 -- Hydraulic Pressure Sensor2/RConn1
  Hydraulic Pressure Sensor1/LConn1 -- hydro_check_valve2/RConn1 -- inverse shuttle valve/LConn2 -- Hydraulic Pressure Sensor4/RConn1 -- B/RConn1
  Hydraulic Pressure Sensor2/LConn1 -- hydro_check_valve1/RConn1 -- inverse shuttle valve/LConn1 -- Hydraulic Pressure Sensor4/LConn1 -- A/RConn1
  hydro_check_valve1/LConn1 -- Hydraulic Flow Rate Sensor/RConn2 -- hydro_check_valve2/LConn1

== system hdv_hydroelectropowertrain_model/PR776_powertrain/Hydrostatic_powertrain/driveline_RD2/vd_ctrl_motor_RD ==
  vd_ref : Inport
  Linear swashplate ctrl2 : linear_swashplate_ctrl_lib/Linear swashplate ctrl  Commented=on  a12=1 1/s  b2=1 1/m/s  k1=100 m  k2=20.5 m  N=5 m  kv=20  xv_specify=off  xv_priority=None  xv=0 m  xv_nominal_specify=off  xv_nominal_unit=m  xv_nominal_value=1  D1_specify=off  D1_priority=None  D1=0  D1_nominal_specify=off  D1_nominal_unit=1  D1_nominal_value=1  D2_specify=off  D2_priority=None  D2=0  D2_nominal_specify=off  D2_nominal_unit=1  D2_nominal_value=1
      settings: InternalSimscapePortConfiguration="{\"Bottom\":[],\"Left\":[{\"id\":\"D_ref\",\"label\":\"Dref\",\"type\":\"input\"}],\"Right\":[{\"id\":\"Dout\",\"label\":\"Dout\",\"type\":\"output\"}],\"Top\":[]}"
  PS-Simulink Converter : nesl_utility/PS-Simulink Converter  PhysicalDomain=network_engine_domain  SubClassName=ps_output  LeftPortType=input  RightPortType=output  PseudoPeriodic=off  Frequencies=[]  VectorFormat=1-D array  Unit=inherit  AffineConversion=off
  Scope : Scope  NumInputPorts=2
  Simulink-PS Converter3 : nesl_utility/Simulink-PS Converter  Commented=on  PhysicalDomain=network_engine_domain  SubClassName=ps_input  LeftPortType=input  RightPortType=output  PseudoPeriodic=off  Frequencies=[]  NoiseDistribution=none  NoiseParameters=[]  Unit=1  AffineConversion=off  FilteringAndDerivatives=provide  SimscapeFilterOrder=1  InputFilterTimeConstant=0.001  UdotUserProvided=0
  hose3 : Subsystem
  servo motor LD : Subsystem
  vd : PMIOPort  Side=Right
  pS : PMIOPort  Port=2  Side=Left
  pT : PMIOPort  Port=3  Side=Left
  wires:
  PS-Simulink Converter/1 -> Scope/2
  vd_ref/1 -> servo motor LD/1(displacement reference pu), Simulink-PS Converter3/1, Scope/1
  connections:
  vd/RConn1 -- PS-Simulink Converter/LConn1 -- servo motor LD/RConn1
  Simulink-PS Converter3/RConn1 -- Linear swashplate ctrl2/LConn1
  pT/RConn1 -- hose3/LConn2
  pS/RConn1 -- hose3/LConn1
  hose3/RConn1 -- servo motor LD/LConn1
  hose3/RConn2 -- servo motor LD/LConn2

== system hdv_hydroelectropowertrain_model/PR776_powertrain/Hydrostatic_powertrain/driveline_RD2/vd_ctrl_pump_RD ==
  vd_ref : Inport
  Linear swashplate ctrl2 : linear_swashplate_ctrl_lib/Linear swashplate ctrl  Commented=on  a12=1 1/s  b2=1 1/m/s  k1=100 m  k2=20.5 m  N=5 m  kv=20  xv_specify=off  xv_priority=None  xv=0 m  xv_nominal_specify=off  xv_nominal_unit=m  xv_nominal_value=1  D1_specify=off  D1_priority=None  D1=0  D1_nominal_specify=off  D1_nominal_unit=1  D1_nominal_value=1  D2_specify=off  D2_priority=None  D2=0  D2_nominal_specify=off  D2_nominal_unit=1  D2_nominal_value=1
      settings: InternalSimscapePortConfiguration="{\"Bottom\":[],\"Left\":[{\"id\":\"D_ref\",\"label\":\"Dref\",\"type\":\"input\"}],\"Right\":[{\"id\":\"Dout\",\"label\":\"Dout\",\"type\":\"output\"}],\"Top\":[]}"
  Simulink-PS Converter3 : nesl_utility/Simulink-PS Converter  Commented=on  PhysicalDomain=network_engine_domain  SubClassName=ps_input  LeftPortType=input  RightPortType=output  PseudoPeriodic=off  Frequencies=[]  NoiseDistribution=none  NoiseParameters=[]  Unit=1  AffineConversion=off  FilteringAndDerivatives=provide  SimscapeFilterOrder=1  InputFilterTimeConstant=0.001  UdotUserProvided=0
  hose3 : Subsystem
  servo pump RD : Subsystem
  vd : PMIOPort  Side=Right
  pS : PMIOPort  Port=2  Side=Left
  pT : PMIOPort  Port=3  Side=Left
  wires:
  vd_ref/1 -> Simulink-PS Converter3/1, servo pump RD/1(displacement reference pu)
  connections:
  Simulink-PS Converter3/RConn1 -- Linear swashplate ctrl2/LConn1
  pT/RConn1 -- hose3/LConn2
  pS/RConn1 -- hose3/LConn1
  servo pump RD/LConn1 -- hose3/RConn1
  servo pump RD/LConn2 -- hose3/RConn2
  servo pump RD/RConn1 -- vd/RConn1

== system hdv_hydroelectropowertrain_model/PR776_powertrain/electrical_main_drive_train/LithiumIonBattery/lithium ion cell analytical ocv ==
  Electrical Reference : fl_lib/Electrical/Electrical Elements/Electrical Reference
  PS Constant : fl_lib/Physical Signals/Sources/PS Constant  constant=298.15 K
  PS-Simulink Converter2 : nesl_utility/PS-Simulink Converter  PhysicalDomain=network_engine_domain  SubClassName=ps_output  LeftPortType=input  RightPortType=output  PseudoPeriodic=off  Frequencies=[]  VectorFormat=1-D array  Unit=inherit  AffineConversion=off
  PS-Simulink Converter3 : nesl_utility/PS-Simulink Converter  PhysicalDomain=network_engine_domain  SubClassName=ps_output  LeftPortType=input  RightPortType=output  PseudoPeriodic=off  Frequencies=[]  VectorFormat=1-D array  Unit=inherit  AffineConversion=off
  PS-Simulink Converter4 : nesl_utility/PS-Simulink Converter  PhysicalDomain=network_engine_domain  SubClassName=ps_output  LeftPortType=input  RightPortType=output  PseudoPeriodic=off  Frequencies=[]  VectorFormat=1-D array  Unit=inherit  AffineConversion=off
  lithium-ion battery with analytical OCV : lithium_ion_cell_lib/lithium-ion Cell with analytical OCV  Qcell=Q A*hr  N=Ncell  E_1=E_1 V  E0=E0 V  E1=E1 V  E2=E2 V  E3=E3 V  Elog=Elog V  R0=R0 Ohm  R1=R1 Ohm  C1=C1 F  M=M V  alpha=alpha  u_specify=off  u_priority=High  u=Vdc V  u_nominal_specify=off  u_nominal_unit=V  u_nominal_value=1  u_ocv_specify=off  u_ocv_priority=High  u_ocv=Vdc V  u_ocv_nominal_specify=off  u_ocv_nominal_unit=V  u_ocv_nominal_value=1  icell_specify=on  icell_priority=High  icell=0 A  icell_nominal_specify=off  icell_nominal_unit=A  icell_nominal_value=1  i_r1_specify=off  i_r1_priority=None  i_r1=0 A  i_r1_nominal_specify=off  i_r1_nominal_unit=A  i_r1_nominal_value=1  z_specify=on  z_priority=High  z=soc_init  z_nominal_specify=off  z_nominal_unit=1  z_nominal_value=1  h_specify=off  h_priority=High  h=0  h_nominal_specify=off  h_nominal_unit=1  h_nominal_value=1
      settings: InternalSimscapePortConfiguration="{\"Bottom\":[],\"Left\":[{\"id\":\"T\",\"label\":\"T\",\"type\":\"input\"}],\"Right\":[{\"id\":\"u_p\",\"label\":\"u+\",\"type\":\"foundation.electrical.electrical\"},{\"id\":\"u_n\",\"label\":\"u-\",\"type\":\"foundation.electrical.electrical\"},{\"id\":\"z_out\",\"label\":\"SOC\",\"type\":\"output\"},{\"id\":\"i_r1_out\",\"label\":\"i_r1\",\"type\":\"output\"},{\"id\":\"h_out\",\"label\":\"hysteresis\",\"type\":\"output\"}],\"Top\":[]}"
  U+ : PMIOPort  Side=Right
  U- : PMIOPort  Port=2  Side=Right
  tag scope: hysteresis=global, icell=global, soc_battery=global
  wires:
  PS-Simulink Converter3/1 -> [soc_battery]  "SOC*"
  PS-Simulink Converter2/1 -> [icell]  "icell"
  PS-Simulink Converter4/1 -> [hysteresis]  "h(t)"
  connections:
  lithium-ion battery with analytical OCV/LConn1 -- PS Constant/RConn1
  lithium-ion battery with analytical OCV/RConn1 -- U+/RConn1
  Electrical Reference/LConn1 -- U-/RConn1 -- lithium-ion battery with analytical OCV/RConn2
  lithium-ion battery with analytical OCV/RConn3 -- PS-Simulink Converter3/LConn1
  lithium-ion battery with analytical OCV/RConn4 -- PS-Simulink Converter2/LConn1
  lithium-ion battery with analytical OCV/RConn5 -- PS-Simulink Converter4/LConn1

== system hdv_hydroelectropowertrain_model/PR776_powertrain/electrical_main_drive_train/dc//dc/iin_ref ==
  current_reference : Subsystem
  iout_ref : Outport
  wires:
  current_reference/1(iin_ref) -> iout_ref/1

== system hdv_hydroelectropowertrain_model/PR776_powertrain/electrical_main_drive_train/dc//dc/iout_ref ==
  current_reference : Subsystem
  iout_ref : Outport
  wires:
  current_reference/1(iout_ref) -> iout_ref/1

== system hdv_hydroelectropowertrain_model/PR776_powertrain/electrical_main_drive_train/dc//dc/sampling_i_filter1 ==
  in : Inport
  1/Ti3 : Gain  Gain=1/150  OutDataTypeStr=double  SaturateOnIntegerOverflow=on  ParamDataTypeStr=Inherit: Same as input
  Saturation : Saturate  UpperLimit=1  LowerLimit=0  OutDataTypeStr=double
  Zero-Order Hold2 : ZeroOrderHold  SampleTime=tsample
  out_pu : Outport
  wires:
  in/1 -> 1/Ti3/1
  1/Ti3/1 -> Saturation/1
  Saturation/1 -> Zero-Order Hold2/1
  Zero-Order Hold2/1 -> out_pu/1

== system hdv_hydroelectropowertrain_model/PR776_powertrain/electrical_main_drive_train/dc//dc/sampling_v_filter1 ==
  in : Inport
  1/Ti3 : Gain  Gain=1/850  OutDataTypeStr=double  SaturateOnIntegerOverflow=on  ParamDataTypeStr=Inherit: Same as input
  Saturation : Saturate  UpperLimit=1  LowerLimit=0  OutDataTypeStr=double
  Zero-Order Hold2 : ZeroOrderHold  SampleTime=tsample
  out_pu : Outport
  wires:
  Zero-Order Hold2/1 -> out_pu/1
  1/Ti3/1 -> Saturation/1
  in/1 -> 1/Ti3/1
  Saturation/1 -> Zero-Order Hold2/1

== system hdv_hydroelectropowertrain_model/PR776_powertrain/electrical_main_drive_train/dc//dc/sampling_v_filter2 ==
  in : Inport
  1/Ti3 : Gain  Gain=1/850  OutDataTypeStr=double  SaturateOnIntegerOverflow=on  ParamDataTypeStr=Inherit: Same as input
  Saturation : Saturate  UpperLimit=1  LowerLimit=0  OutDataTypeStr=double
  Zero-Order Hold2 : ZeroOrderHold  SampleTime=tsample
  out_pu : Outport
  wires:
  in/1 -> 1/Ti3/1
  1/Ti3/1 -> Saturation/1
  Zero-Order Hold2/1 -> out_pu/1
  Saturation/1 -> Zero-Order Hold2/1

== system hdv_hydroelectropowertrain_model/PR776_powertrain/electrical_main_drive_train/dc//dc/sampling_v_filter3 ==
  in : Inport
  1/Ti3 : Gain  Gain=1/150  OutDataTypeStr=double  SaturateOnIntegerOverflow=on  ParamDataTypeStr=Inherit: Same as input
  Saturation : Saturate  UpperLimit=1  LowerLimit=0  OutDataTypeStr=double
  Zero-Order Hold2 : ZeroOrderHold  SampleTime=tsample
  out_pu : Outport
  wires:
  Saturation/1 -> Zero-Order Hold2/1
  Zero-Order Hold2/1 -> out_pu/1
  1/Ti3/1 -> Saturation/1
  in/1 -> 1/Ti3/1

== system hdv_hydroelectropowertrain_model/PR776_powertrain/electrical_main_drive_train/dc//dc/sampling_v_filter4 ==
  in : Inport
  1/Ti3 : Gain  Gain=1/300  OutDataTypeStr=double  SaturateOnIntegerOverflow=on  ParamDataTypeStr=Inherit: Same as input
  Saturation : Saturate  UpperLimit=1  LowerLimit=0  OutDataTypeStr=double
  Zero-Order Hold2 : ZeroOrderHold  SampleTime=tsample
  out_pu : Outport
  wires:
  in/1 -> 1/Ti3/1
  1/Ti3/1 -> Saturation/1
  Zero-Order Hold2/1 -> out_pu/1
  Saturation/1 -> Zero-Order Hold2/1

== system hdv_hydroelectropowertrain_model/PR776_powertrain/electrical_main_drive_train/dc//dc/sampling_v_filter5 ==
  in : Inport
  1/Ti3 : Gain  Gain=1/300  OutDataTypeStr=double  SaturateOnIntegerOverflow=on  ParamDataTypeStr=Inherit: Same as input
  Saturation : Saturate  UpperLimit=1  LowerLimit=0  OutDataTypeStr=double
  Zero-Order Hold2 : ZeroOrderHold  SampleTime=tsample
  out_pu : Outport
  wires:
  Saturation/1 -> Zero-Order Hold2/1
  in/1 -> 1/Ti3/1
  1/Ti3/1 -> Saturation/1
  Zero-Order Hold2/1 -> out_pu/1

== system hdv_hydroelectropowertrain_model/PR776_powertrain/electrical_main_drive_train/dc//dc/vi ctrl ==
  iout : Inport
  vout : Inport  Port=2
  vout_ref : Inport  Port=3
  iout_ref : Inport  Port=4
  iin : Inport  Port=5
  iin_ref : Inport  Port=6
  Iin Ctrl : Subsystem
  Iout Ctrl : Subsystem
  Min : MinMax  Inputs=3
  Sum : Sum  Inputs=++|
  Unit Delay2 : UnitDelay  SampleTime=tsample  HasFrameUpgradeWarning=on
  Vout Ctrl : Subsystem
  iin_ref/iin : Scope  NumInputPorts=2
  iout_ref/iout : Scope  NumInputPorts=2
  vout_ref/vout : Scope  NumInputPorts=2
  phase_out : Outport
  wires:
  Unit Delay2/1 -> phase_out/1
  iout/1 -> iout_ref/iout/2, Iout Ctrl/2(iout)
  vout_ref/1 -> vout_ref/vout/1, Vout Ctrl/1(vout_ref)
  vout/1 -> Sum/1, vout_ref/vout/2, Vout Ctrl/2(vout)
  iout_ref/1 -> iout_ref/iout/1, Iout Ctrl/1(iout_ref)
  Iout Ctrl/1(ctrli_out) -> Sum/2
  Sum/1 -> Min/2
  Vout Ctrl/1(ctrlv_out) -> Min/1
  Min/1 -> Unit Delay2/1
  Iin Ctrl/1(ctrli_out) -> Min/3
  iin_ref/1 -> Iin Ctrl/1(iin_ref), iin_ref/iin/1
  iin/1 -> Iin Ctrl/2(iin), iin_ref/iin/2

== system hdv_hydroelectropowertrain_model/PR776_powertrain/electrical_main_drive_train/dc//dc/vout_ref ==
  voltage_reference : Subsystem
  vout_ref : Outport
  wires:
  voltage_reference/1(vout_ref) -> vout_ref/1
